simulink model "simulator"  (R2016b)
settings: Solver=ode23tb  StartTime=0.0  StopTime=20  RelTol=1e-4  EnableMultiTasking=on
settings Model: Creator=ROMERO_VELAZQUEZ  LastModifiedBy=erick
settings SolverCC: SolverResetMethod=Robust
settings DataIOCC: LimitDataPoints=on  SaveFormat=Array  SignalLoggingSaveFormat=ModelDataLogs
settings OptimizationCC: ExpressionDepthLimit=2147483647  LifeSpan=inf
settings DebuggingCC: UnderspecifiedInitializationDetection=Classic  MergeDetectMultiDrivingBlocksExec=none  SolverPrmCheckMsg=warning  FcnCallInpInsideContextMsg=warning  StateNameClashWarn=warning  SFUnexpectedBacktrackingDiag=warning  SFNoUnconditionalDefaultTransitionDiag=warning  SFExecutionAtInitializationDiag=none
settings HardwareCC: ProdBitPerPointer=32  ProdBitPerSizeT=32  ProdBitPerPtrDiffT=32  ProdLargestAtomicFloat=None  ProdIntDivRoundTo=Undefined  ProdEndianess=Unspecified  ProdWordSize=32  ProdHWDeviceType=32-bit Generic
settings ModelReferenceCC: PropagateSignalLabelsOutOfModel=off
settings GRTTargetCC: TargetLangStandard=C89/C90 (ANSI)  GeneratePreprocessorConditionals=Disable all  CombineOutputUpdateFcns=off  GRTInterface=on
settings ConfigComp: CovMetricSettings=dw  CovHtmlReporting=on  CovSaveCumulativeToWorkspaceVar=on  CovSaveSingleToWorkspaceVar=on  CovExternalEMLEnable=off  CovSFcnEnable=off

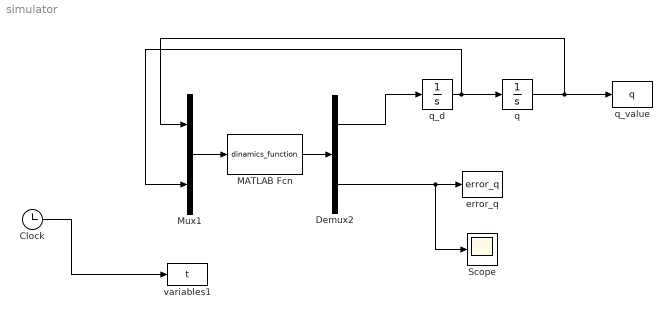
== system simulator ==
  Clock : Clock
  Demux2 : Demux  Outputs=[3,3]
  MATLAB Fcn : MATLABFcn  MATLABFcn=dinamics_function  OutputDimensions=6
  Mux1 : Mux  Inputs=2
  Scope : Scope
  error_q : ToWorkspace  VariableName=error_q  SampleTime=-1
  q : Integrator  InitialCondition=[-1.9;-1.9;-2.0]
  q_d : Integrator  InitialCondition=[-7.87;-6.7;.2]
  q_value : ToWorkspace  VariableName=q  SampleTime=-1
  variables1 : ToWorkspace  VariableName=t  SampleTime=-1
  wires:
  Mux1/1 -> MATLAB Fcn/1
  MATLAB Fcn/1 -> Demux2/1
  Demux2/1 -> q_d/1
  Clock/1 -> variables1/1
  q/1 -> q_value/1, Mux1/1
  q_d/1 -> Mux1/2, q/1
  Demux2/2 -> Scope/1, error_q/1
